simulink model "esboco_simulink"  (R2017b)
settings: Solver=VariableStepAuto  StartTime=0.0  StopTime=10.0  RelTol=1e-3
settings Model: Creator=Luís Miranda  LastModifiedBy=Luís Miranda

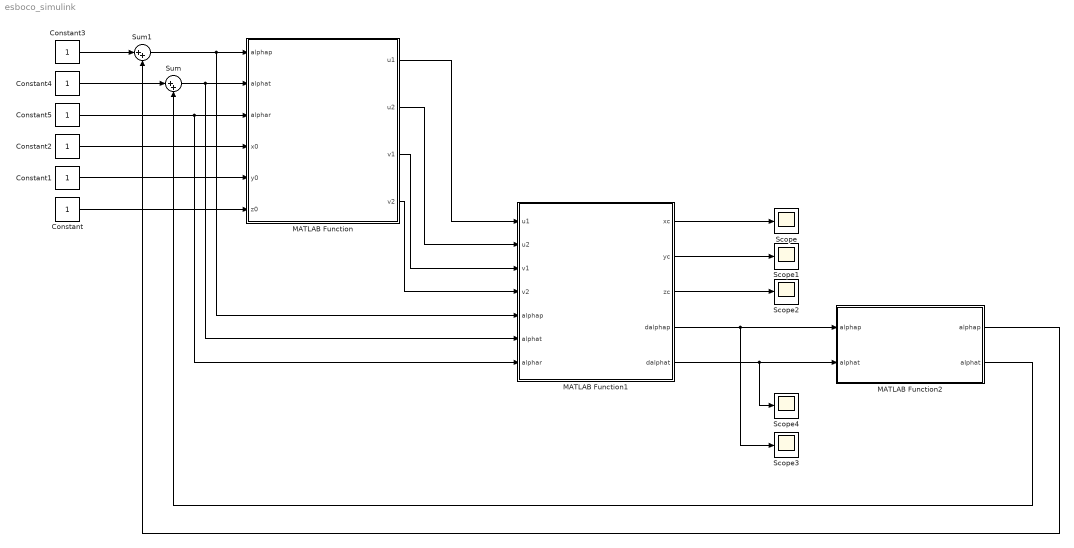
== system esboco_simulink ==
  Constant{,1..5} (6 alike) : Constant
  MATLAB Function : MATLAB Function  TreatAsAtomicUnit=on
  MATLAB Function1 : MATLAB Function  TreatAsAtomicUnit=on
  MATLAB Function2 : MATLAB Function  TreatAsAtomicUnit=on
  Scope{,1..4} (5 alike) : Scope
  Sum : Sum  Inputs=|++
  Sum1 : Sum  Inputs=|++
  wires:
  MATLAB Function/1(u1) -> MATLAB Function1/1(u1)
  MATLAB Function/2(u2) -> MATLAB Function1/2(u2)
  MATLAB Function/3(v1) -> MATLAB Function1/3(v1)
  MATLAB Function/4(v2) -> MATLAB Function1/4(v2)
  Constant2/1 -> MATLAB Function/4(x0)
  Constant1/1 -> MATLAB Function/5(y0)
  Constant/1 -> MATLAB Function/6(z0)
  Constant5/1 -> MATLAB Function/3(alphar), MATLAB Function1/7(alphar)
  Constant4/1 -> Sum/1
  Constant3/1 -> Sum1/1
  Sum1/1 -> MATLAB Function1/5(alphap), MATLAB Function/1(alphap)
  Sum/1 -> MATLAB Function1/6(alphat), MATLAB Function/2(alphat)
  MATLAB Function1/1(xc) -> Scope/1
  MATLAB Function1/2(yc) -> Scope1/1
  MATLAB Function1/3(zc) -> Scope2/1
  MATLAB Function1/4(dalphap) -> MATLAB Function2/1("alphap "), Scope3/1
  MATLAB Function1/5(dalphat) -> Scope4/1, MATLAB Function2/2("alphat ")
  MATLAB Function2/1(alphap) -> Sum1/2
  MATLAB Function2/2(alphat) -> Sum/2

== matlab function esboco_simulink/MATLAB Function1 ==
  data: xc output; u1 input; yc output; u2 input; v1 input; v2 input; zc output; alphap input; alphat input; alphar input; dalphap output; dalphat output
function [xc, yc, zc, dalphap, dalphat]  = camera2real(u1, u2, v1, v2, alphap, alphat, alphar)

%atribuir valor de f
f=664;

%atribuir valor de L
L=1;

xc=(((-f*cos(alphap-alphar)-u2*sin(alphap-alphar))*((f^2)*cos(alphap-alphar)*sin(alphap-alphar)+f*(cos(alphap-alphar)^2)*(u1+u2)-u1)-sin(alphap-alphar)*cos(alphap-alphar)*u1*u2)*L)/(f*(f*sin(alphap-alphar)+u2*cos(alphap-alphar))*(u1-u2));

yc=-(((f^2)*sin(2*(alphap-alphar))+f*((2*(cos(alphap-alphar)^2))-1)*(u1+u2)-sin(2*(alphap-alphar))*u1*u2)*L)/(2*f*(u1-u2));

zc=-(((f^2)*sin(2*(alphat))+f*((2*(cos(alphat)^2))-1)*(v1+v2)-sin(2*(alphat))*v1*v2)*L)/(2*f*(v1-v2));

dalphap=atan(yc,xc)-alphar

dalphat=atan(zc,sqrt((xc^2)+(yc^2)))

== matlab function esboco_simulink/MATLAB Function ==
  data: alphap input; u1 output; alphat input; alphar input; x0 input; y0 input; z0 input; u2 output; v1 output; v2 output
function [u1, u2, v1, v2] = object2image(alphap, alphat, alphar, x0, y0, z0)

%atribuir valor de f
f=664;

%atribuir valor de L
L=1;

v1=f*(sin(alphap-alphar)*x-cos(alphap-alphar)*z+cos(alphap-alphar)*(L/2))/(-cos(alphap-alphar)*x-sin(alphap-alphar)*z+sin(alphap-alphar)*(L/2));

v2=f*(sin(alphap-alphar)*x-cos(alphap-alphar)*z-cos(alphap-alphar)*(L/2))/(-cos(alphap-alphar)*x-sin(alphap-alphar)*z-sin(alphap-alphar)*(L/2));

== matlab function esboco_simulink/MATLAB Function2 ==
  data: alphap input; alphap output; alphat input; alphat output
function [alphap, alphat] = servosystem(alphap, alphat)

;
